simulink model "TOLQRClosedLoopHW2023"  (R2023a)
settings: Solver=FixedStepDiscrete  StartTime=0.0  StopTime=4  FixedStep=0.001  RelTol=1e-3  EnableMultiTasking=on
values from neighbouring files (symbols this model uses):
  x0 = [-pi/2;0;0;0]    [MAIN.m]    (also in MAIN_HW.m; fitParams.m = [-pi/2; 0; 0; 0])
undefined symbols (not defined in the file or in its folder): dC, DiscIntNeverNeededParam, HIL
libraries: quarc_library x3, simulink x1, eeGeneralControl x1
settings Model: ExtModeTrigType=signal  ExtModeTrigDuration=10000  ExtModeTrigDirection=either  ExtModeTrigLevel=0.500000  Creator=colegiusto  LastModifiedBy=colegiusto
settings SolverCC: PositivePriorityOrder=on
settings RTWCC: Description=QUARC Win64 Target Using Toolchain  SystemTargetFile=quarc_win64.tlc  Toolchain=QUARC win64 | nmake (64-bit Windows)  BuildConfiguration=Faster Runs
settings STFCustomTargetCC: TargetLangStandard=C89/C90 (ANSI)  SystemTargetFile=quarc_win64.tlc
settings GRTTargetCC: TargetLangStandard=C89/C90 (ANSI)  ParMdlRefBuildCompliant=off  CompOptLevelCompliant=off  CombineOutputUpdateFcns=off  MatFileLogging=off  CPPClassGenCompliant=off  GRTInterface=on  ExtMode=on  ExtModeMexFile=quarc_comm

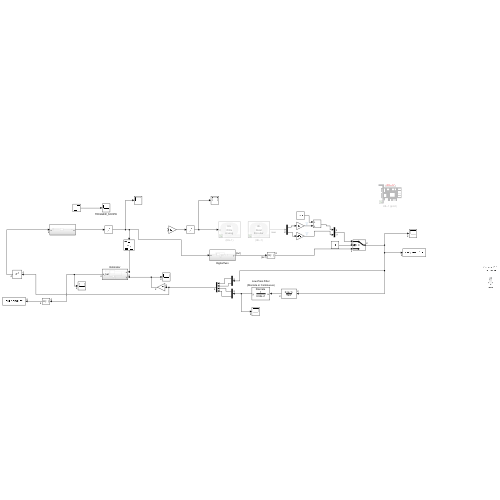
[thumbnail: Simulink's stored preview of the top-level diagram]
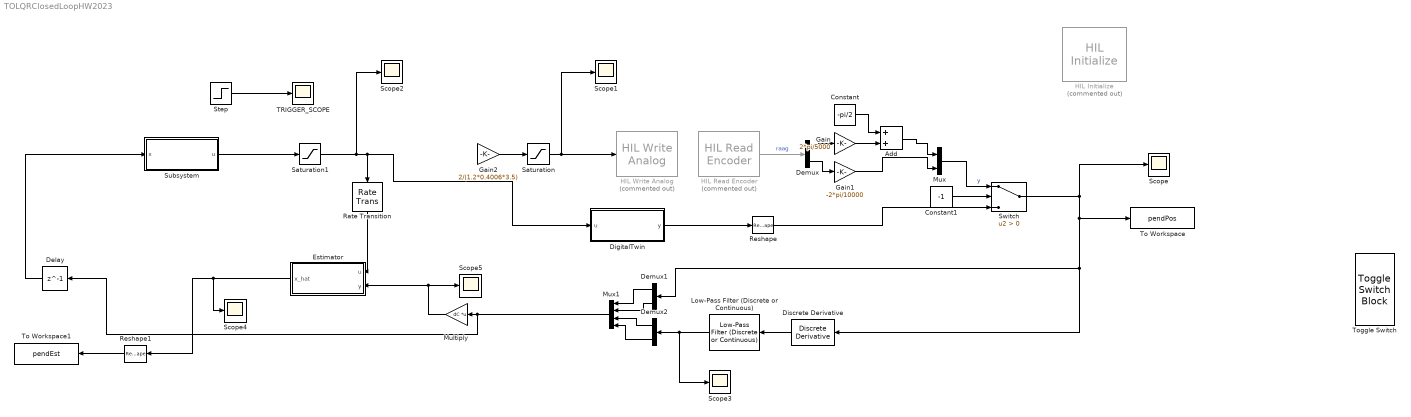
== system TOLQRClosedLoopHW2023 ==
  Add : Sum
  Constant : Constant  Value=-pi/2
  Constant1 : Constant  Value=-1
  Delay : Delay  DelayLength=1  InitialCondition=x0
  Demux : Demux  Outputs=2
  Demux1 : Demux  Outputs=2
  Demux2 : Demux  Outputs=2
  DigitalTwin : Subsystem
  Discrete Derivative : simulink/Discrete/Discrete Derivative  gainval=1.0  ICPrevScaledInput=x0(1:2)/0.001  OutMin=[]  OutMax=[]  OutDataType=fixdt(1, 16)  OutScaling=2^-10  DoSatur=off
  Estimator : Subsystem
  Gain : Gain  Gain=2*pi/5000
  Gain1 : Gain  Gain=-2*pi/10000
  Gain2 : Gain  Gain=2/(1.2*0.4006*3.5)
  HIL Initialize : quarc_library/Data Acquisition/Generic/Configuration/HIL Initialize  Commented=on  object_name=HIL-1  board_type=q4  board_number=0  board_options=""  exclusive=off  active=on  hardware_clocks=[0:1]  clock_modes=[0 0]  initial_clock_frequencies=[]  set_clock_params_at_start=on  set_clock_params_at_switch_in=off  set_clock_frequencies_at_start=off  set_clock_frequencies_at_switch_in=off  analog_input_channels=[0:3]  analog_input_configurations=[]  analog_input_maximums=10  analog_input_minimums=-10  set_analog_input_params_at_start=off  set_analog_input_params_at_switch_in=off  analog_output_channels=[0:3]  analog_output_maximums=[10]  analog_output_minimums=[-10]  initial_analog_outputs=[0]  final_analog_outputs=[0]  watchdog_analog_outputs=0  set_analog_output_params_at_start=on  set_analog_output_params_at_switch_in=off  set_analog_outputs_at_start=on  set_analog_outputs_at_switch_in=off  set_analog_outputs_at_terminate=on  set_analog_outputs_at_switch_out=off  set_analog_outputs_on_watchdog=off  digital_input_channels=[]  digital_output_channels=[]  digital_output_configuration=[]  initial_digital_outputs=[1]  final_digital_outputs=[1]  watchdog_digital_outputs=[2]  set_digital_output_params_at_start=off  set_digital_output_params_at_switch_in=off  set_digital_outputs_at_start=on  set_digital_outputs_at_switch_in=off  set_digital_outputs_at_terminate=on  set_digital_outputs_at_switch_out=off  set_digital_outputs_on_watchdog=off  encoder_channels=[0:3]  quadrature=[4]  encoder_filter_frequency=(1/60e-9)/1  initial_encoder_counts=[0]  set_encoder_params_at_start=on  set_encoder_params_at_switch_in=off  set_encoder_counts_at_start=on  set_encoder_counts_at_switch_in=off  pwm_channels=[]  pwm_modes=[0]  pwm_frequency=(1/60e-9)/1024  pwm_configuration=[]  pwm_alignment=[]  pwm_polarity=[]  pwm_leading_deadband=[]  pwm_trailing_deadband=[]  initial_pwm_outputs=[0]  final_pwm_outputs=[0]  watchdog_pwm_outputs=[]  set_pwm_params_at_start=on  set_pwm_params_at_switch_in=off  set_pwm_outputs_at_start=on  set_pwm_outputs_at_switch_in=off  set_pwm_outputs_at_terminate=on  set_pwm_outputs_at_switch_out=off  set_pwm_outputs_on_watchdog=off  other_output_channels=[]  initial_other_outputs=[]  final_other_outputs=[]  watchdog_other_outputs=[]  set_other_outputs_at_start=off  set_other_outputs_at_switch_in=off  set_other_outputs_at_terminate=off  set_other_outputs_at_switch_out=off  set_other_outputs_on_watchdog=off
  HIL Read Encoder : quarc_library/Data Acquisition/Generic/Immediate I//O/HIL Read Encoder  Commented=on  object_name=HIL-1  channels=[0:1]  sample_time=0.001  active=on  vector_output=on  data_type_mode=Inherit via back propagation  data_type=double
  HIL Write Analog : quarc_library/Data Acquisition/Generic/Immediate I//O/HIL Write Analog  Commented=on  object_name=HIL-1  channels=0  sample_time=0.001  active=off  vector_input=off
  Low-Pass Filter (Discrete or Continuous) : eeGeneralControl/Low-Pass Filter (Discrete or Continuous)  K=1  T=0.04  B=inf  A=-inf  init_option=Inherited from block input  x0=0  Ts=-1
  Multiply : Gain  Gain=dC  Multiplication=Matrix(K*u)
  Mux : Mux  Inputs=2
  Mux1 : Mux
  Rate Transition : RateTransition  OutPortSampleTime=0.001
  Reshape : Reshape
  Reshape1 : Reshape
  Saturation : Saturate  UpperLimit=1  LowerLimit=-1
  Saturation1 : Saturate  UpperLimit=2  LowerLimit=-2
  Scope{,1..5} (6 alike) : Scope
  Step : Step  Time=0.001  SampleTime=0
  Subsystem : Subsystem
  Switch : Switch  Criteria=u2 > Threshold  SaturateOnIntegerOverflow=off  InputSameDT=off
  TRIGGER_SCOPE : Scope
  To Workspace : ToWorkspace  VariableName=pendPos  SaveFormat=Structure With Time  SampleTime=-1
  To Workspace1 : ToWorkspace  VariableName=pendEst  SaveFormat=Structure With Time  SampleTime=-1
  Toggle Switch : ToggleSwitchBlock
      settings: Values={{'Sim', 'Hardware'}, [-1 1]}
  wires:
  HIL Read Encoder/1 -> Demux/1  "raag"
  Step/1 -> TRIGGER_SCOPE/1
  Demux/2 -> Gain1/1
  Demux/1 -> Gain/1
  Gain1/1 -> Mux/2
  Gain2/1 -> Saturation/1
  Add/1 -> Mux/1
  Gain/1 -> Add/2
  Constant/1 -> Add/1
  Demux1/1 -> Mux1/1
  Demux1/2 -> Mux1/2
  Demux2/1 -> Mux1/3
  Demux2/2 -> Mux1/4
  Saturation/1 -> Scope1/1, HIL Write Analog/1
  Rate Transition/1 -> Estimator/1(u)
  Estimator/1(x_hat) -> Reshape1/1, Scope4/1
  DigitalTwin/1(y) -> Reshape/1
  Delay/1 -> Subsystem/1(x)
  Reshape1/1 -> To Workspace1/1
  Mux1/1 -> Delay/1, Multiply/1
  Multiply/1 -> Estimator/2(y), Scope5/1
  Reshape/1 -> Switch/3
  Mux/1 -> Switch/1  "y"
  Switch/1 -> Scope/1, Demux1/1, Discrete Derivative/1, To Workspace/1
  Constant1/1 -> Switch/2
  Subsystem/1(u) -> Saturation1/1
  Discrete Derivative/1 -> Low-Pass Filter (Discrete or Continuous)/1
  Saturation1/1 -> Rate Transition/1, DigitalTwin/1(u), Scope2/1
  Low-Pass Filter (Discrete or Continuous)/1 -> Scope3/1, Demux2/1

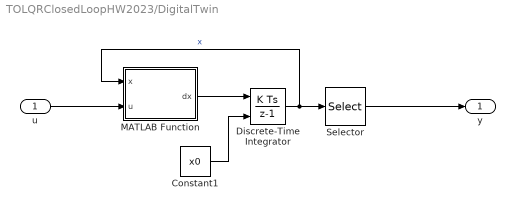
== system TOLQRClosedLoopHW2023/DigitalTwin ==
  u : Inport
  Constant1 : Constant  Value=x0  VectorParams1D=off
  Discrete-Time Integrator : DiscreteIntegrator  InitialConditionSource=external  SampleTime=-1  ICPrevOutput=DiscIntNeverNeededParam  ICPrevScaledInput=DiscIntNeverNeededParam
  MATLAB Function : MATLAB Function  TreatAsAtomicUnit=on
  Selector : Selector  InputPortWidth=4  IndexOptions=Index vector (dialog)  Indices=[1 2]  OutputSizes=1
  y : Outport
  wires:
  Discrete-Time Integrator/1 -> Selector/1, MATLAB Function/1(x)  "x"
  Constant1/1 -> Discrete-Time Integrator/2
  MATLAB Function/1(dx) -> Discrete-Time Integrator/1
  u/1 -> MATLAB Function/2(u)
  Selector/1 -> y/1

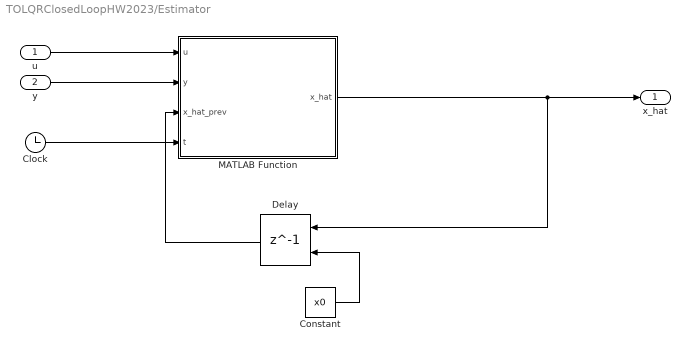
== system TOLQRClosedLoopHW2023/Estimator ==
  u : Inport
  y : Inport  Port=2
  Clock : Clock
  Constant : Constant  Value=x0  VectorParams1D=off
  Delay : Delay  DelayLength=1  InitialConditionSource=Input port  InitialCondition=[0; 0; 0; 0]
      settings: InputPortMap=u0,p4
  MATLAB Function : MATLAB Function  TreatAsAtomicUnit=on
  x_hat : Outport
  wires:
  MATLAB Function/1(x_hat) -> Delay/1, x_hat/1
  y/1 -> MATLAB Function/2(y)
  Delay/1 -> MATLAB Function/3(x_hat_prev)
  Constant/1 -> Delay/2
  u/1 -> MATLAB Function/1(u)
  Clock/1 -> MATLAB Function/4(t)

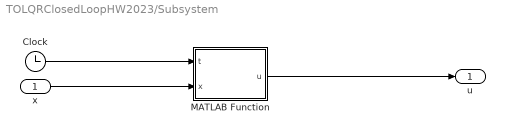
== system TOLQRClosedLoopHW2023/Subsystem ==
  x : Inport
  Clock : Clock
  MATLAB Function : MATLAB Function  TreatAsAtomicUnit=on
  u : Outport
  wires:
  x/1 -> MATLAB Function/2(x)
  Clock/1 -> MATLAB Function/1(t)
  MATLAB Function/1(u) -> u/1

== matlab function TOLQRClosedLoopHW2023/DigitalTwin/MATLAB Function ==
  data: x input; u input; dx output; p parameter
function dx = dyn(x,u,p)
    dx = dynamics(x,u,p);
end

== matlab function TOLQRClosedLoopHW2023/Subsystem/MATLAB Function ==
  data: t input; u output; x input; c parameter
function u = fcn(t,x,c)

u = TOLQRlinearControl(t,x,c);

== matlab function TOLQRClosedLoopHW2023/Estimator/MATLAB Function ==
  data: u input; x_hat output; y input; x_hat_prev input; t input; c parameter
function x_hat = fcn(u, y, x_hat_prev, t, c)

    m = 1+ length(y);

    x_hat = zeros([4 1]);

    % Determine most recent knot point
    index = find(c.t_k > t, 1)-1;
    if t >= c.t_k(end)
        index = length(c.t_k);
        next = index;
        interp = 0;
    else
        next = index + 1;
        interp = (t-c.t_k(index))/(c.t_k(next)-c.t_k(index));
    end



    % Interpolate trajectory reference state
    x_star = c.x_star(:,index)*(1-interp) ... 
        + c.x_star(:,next)*interp;

    % Interpolate trajectory reference input
    u_star = c.u_star(index)*(1-interp)+ ...
        +c.u_star(next)*interp;


    % Pick A,B linearized around knot point
    A = c.A(:,:,index);
    B = c.B(:,:,index);
    
    u_ext = reshape([u-u_star; (y-eye(2,4)*x_star)], [m 1]);
    x_hat_prev = reshape(x_hat_prev, [4 1]);
    
    
    x_hat(:,1) = x_star + A* (x_hat_prev-x_star) + B*u_ext;
